simulink subsystem "Get_Traffic"  (R2022b)
settings: Solver=VariableStepAuto  StartTime=0.0  StopTime=10.0  RelTol=1e-3
libraries: CarMaker4SL x3
settings Model: Creator=user  LastModifiedBy=user

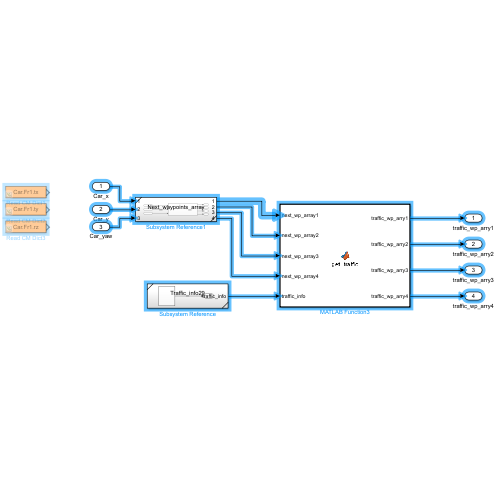
[thumbnail: Simulink's stored preview of the top-level diagram]
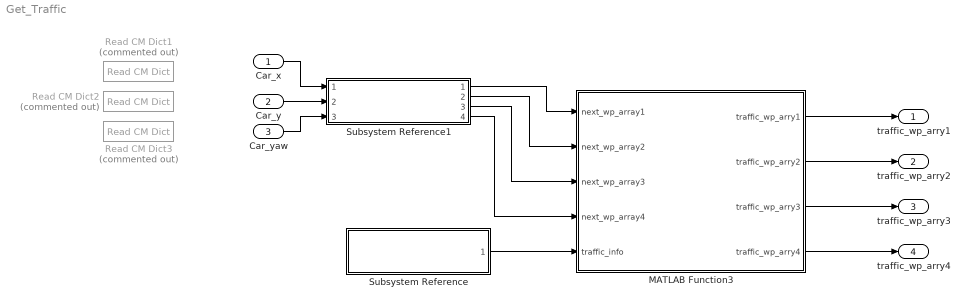
== system Get_Traffic ==
  Car_x : Inport
  Car_y : Inport  Port=2
  Car_yaw : Inport  Port=3
  MATLAB Function3 : MATLAB Function  TreatAsAtomicUnit=on
  Read CM Dict1 : CarMaker4SL/Read CM Dict  Commented=on  xname=Car.Fr1.tx  xsync=off  xstime=Inherited
  Read CM Dict2 : CarMaker4SL/Read CM Dict  Commented=on  xname=Car.Fr1.ty  xsync=off  xstime=Inherited
  Read CM Dict3 : CarMaker4SL/Read CM Dict  Commented=on  xname=Car.Fr1.rz  xsync=off  xstime=Inherited
  Subsystem Reference : Subsystem  ReferencedSubsystem=Traffic_info29
  Subsystem Reference1 : Subsystem  ReferencedSubsystem=Next_waypoints_array
  traffic_wp_arry1 : Outport
  traffic_wp_arry2 : Outport  Port=2
  traffic_wp_arry3 : Outport  Port=3
  traffic_wp_arry4 : Outport  Port=4
  wires:
  MATLAB Function3/4(traffic_wp_arry4) -> traffic_wp_arry4/1
  MATLAB Function3/2(traffic_wp_arry2) -> traffic_wp_arry2/1
  Subsystem Reference1/3 -> MATLAB Function3/3(next_wp_array3)
  Subsystem Reference/1 -> MATLAB Function3/5(traffic_info)
  MATLAB Function3/3(traffic_wp_arry3) -> traffic_wp_arry3/1
  Car_y/1 -> Subsystem Reference1/2
  Car_x/1 -> Subsystem Reference1/1
  Subsystem Reference1/4 -> MATLAB Function3/4(next_wp_array4)
  Subsystem Reference1/2 -> MATLAB Function3/2(next_wp_array2)
  MATLAB Function3/1(traffic_wp_arry1) -> traffic_wp_arry1/1
  Car_yaw/1 -> Subsystem Reference1/3
  Subsystem Reference1/1 -> MATLAB Function3/1(next_wp_array1)

== matlab function Get_Traffic/MATLAB Function3 ==
  settings: updateMethod=DISCRETE  sampleTime=0.05
  data: next_wp_array1 input; next_wp_array2 input; next_wp_array3 input; next_wp_array4 input; traffic_wp_arry1 output size=[1000, 1000]; traffic_info input; traffic_wp_arry2 output; traffic_wp_arry3 output; traffic_wp_arry4 output
function [traffic_wp_arry1, traffic_wp_arry2, traffic_wp_arry3, traffic_wp_arry4] = get_traffic(next_wp_array1, next_wp_array2, next_wp_array3, next_wp_array4, traffic_info)
    num_wp = 10; % 웨이포인트 수
    tolerance = 2; % 트래픽 위치에 대한 오차 허용 범위

    % Initialize traffic waypoints array
    traffic_wp_arry1 = nan(num_wp, 2);
    traffic_wp_arry2 = nan(num_wp, 2);
    traffic_wp_arry3 = nan(num_wp, 2);
    traffic_wp_arry4 = nan(num_wp, 2);

    % 트래픽 정보를 29x3으로 재구성
    traffic_array = reshape(traffic_info, 3, []); % 29개의 트래픽 정보 (x, y, yaw)

    % 트래픽이 있는 웨이포인트 필터링
    for wp_set = 1:4
        if wp_set == 1
            next_wp_array = next_wp_array1;
        elseif wp_set == 2
            next_wp_array = next_wp_array2;
        elseif wp_set == 3
            next_wp_array = next_wp_array3;
        else
            next_wp_array = next_wp_array4;
        end
        
        traffic_wp_array = nan(num_wp, 2);
        
        for i = 1:num_wp
            wp_x = next_wp_array(i, 1);
            wp_y = next_wp_array(i, 2);
            
            % 트래픽 배열에서 각 트래픽 정보와 비교
            for j = 1:size(traffic_array, 1)
                traffic_x = traffic_array(j, 1);
                traffic_y = traffic_array(j, 2);
                
                % 트래픽 위치가 웨이포인트 위치 근처에 있는지 확인 (오차 범위 내)
                if abs(traffic_x - wp_x) <= tolerance && abs(traffic_y - wp_y) <= tolerance
                    traffic_wp_array(i, :) = next_wp_array(i, :); % 트래픽이 있으면 해당 웨이포인트 저장
                    break; % 한 번 트래픽을 찾으면 더 이상 해당 웨이포인트를 확인하지 않음
                end
            end
        end

        % 해당 결과를 각각의 트래픽 웨이포인트 배열에 저장
        if wp_set == 1
            traffic_wp_arry1 = traffic_wp_array;
        elseif wp_set == 2
            traffic_wp_arry2 = traffic_wp_array;
        elseif wp_set == 3
            traffic_wp_arry3 = traffic_wp_array;
        else
            traffic_wp_arry4 = traffic_wp_array;
        end
    end

end
